simulink model "gyroscope_temps_reel"  (R2013a)
settings: Solver=ode3  StartTime=0.0  StopTime=inf  FixedStep=Ts  RelTol=1e-3
values from neighbouring files (symbols this model uses):
  Aobs2 = A2-H2*C2    [speed_w1_estimation.m]
  Bobs2 = [B2 H2]    [speed_w1_estimation.m]
  Cobs2 = [0 1]    [speed_w1_estimation.m]
  Dobs2 = zeros(1,2)    [speed_w1_estimation.m]
  Te = Ts    [speed_w1_estimation.m]
undefined symbols (not defined in the file or in its folder): C0, Kp, Standard_Devices, UDP_Protocol
libraries: etargetslib x13, simulink x2, rtwinlib x2
settings Model: SimulationMode=external  ExtModeTrigDuration=100000  Creator=dumonjon  LastModifiedBy=khennouh
settings DataIOCC: LimitDataPoints=off  SaveFormat=StructureWithTime  SignalLoggingSaveFormat=ModelDataLogs  SaveOutput=off  SignalLogging=off  SaveTime=off
settings OptimizationCC: ExpressionDepthLimit=2147483647  InitFltsAndDblsToZero=on
settings DebuggingCC: FcnCallInpInsideContextMsg=UseLocalSettings  StrictBusMsg=Warning
settings SFSimCC: SimParseCustomCode=off
settings RTWCC: SystemTargetFile=rtwin.tlc  TemplateMakefile=rtwin.tmf  Description=Real-Time Windows Target  ProcessScript=rtwin_make_rtw_hook
settings TargetCC: CodeReplacementLibrary=ANSI_C  IsPILTarget=off  ModelReferenceCompliant=off  CompOptLevelCompliant=off  EnableShiftOperators=on

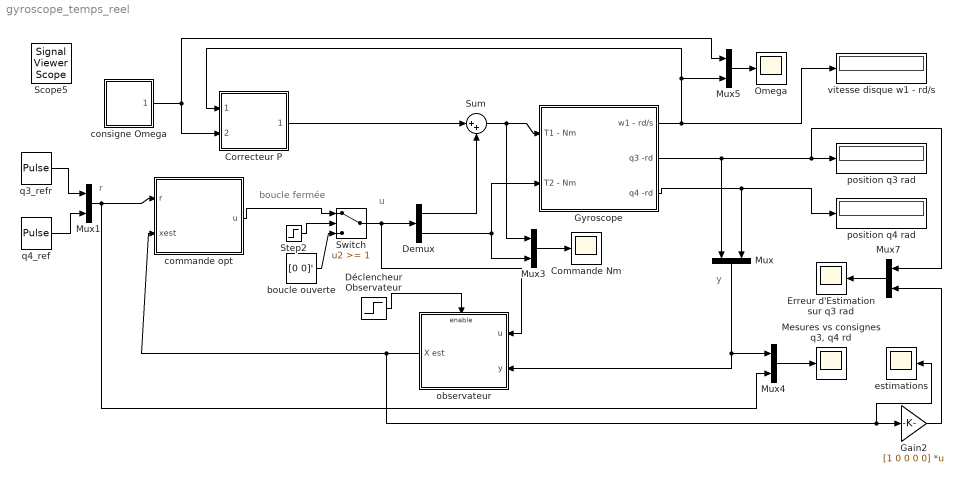
== system gyroscope_temps_reel ==
  note: u
  note: r
  note: y
  note: boucle fermée
  Commande Nm : Scope
      settings: TimeRange=70  YMin=-0.2  YMax=0.5  SaveName=commande
  Correcteur P : Subsystem
  Demux : Demux  Outputs=2
  Déclencheur Observateur : Step  SampleTime=0
  Erreur d'Estimation sur q3 rad : Scope
      settings: TimeRange=70  YMin=-0.6000000000000001  YMax=0.8  SaveName=theta3
  Gain2 : Gain  Gain=[1 0 0 0 0]  Multiplication=Matrix(K*u) (u vector)
  Gyroscope : Subsystem
  "Mesures vs consignes q3, q4 rd" : Scope
      settings: TimeRange=70  YMin=-0.35  YMax=0.35  SaveName=consigne
  Mux{,1,3..5,7} (6 alike) : Mux  Inputs=2
  Omega : Scope
      settings: TimeRange=60  YMin=0  YMax=60  SaveName=omega
  Step2 : Step  Time=15  SampleTime=0
  Sum : Sum  Inputs=|++
  Switch : Switch  Threshold=1
  boucle ouverte : Constant  Value=[0 0]'
  commande opt : Subsystem
  consigne Omega : Subsystem  mask{Omega=42}
  estimations : Scope
      settings: TimeRange=70  YMin=-1.5  YMax=1  SaveName=estimations
  observateur : Subsystem
  position q3 rad : Display
  position q4 rad : Display
  q3_refr : DiscretePulseGenerator  PulseType=Time based  Amplitude=10*pi/180  Period=20  PulseWidth=50  PhaseDelay=20
  q4_ref : DiscretePulseGenerator  PulseType=Time based  Amplitude=10*pi/180  Period=20  PulseWidth=50  PhaseDelay=25
  vitesse disque w1 - rd/s : Display
  Scope5 : SignalViewerScope  IOType=viewer  RefreshTime=0.035000
  wires:
  consigne Omega/1(Cw1 rd/s) -> Correcteur P/2(Cw1 rd/s), Mux5/1
  Demux/2 -> Mux3/2, Gyroscope/2(T2 - Nm)
  Sum/1 -> Gyroscope/1(T1 - Nm), Mux3/1
  Gyroscope/2(q3 -rd) -> Mux/1, position q3 rad/1, Mux7/1
  Gyroscope/3(q4 -rd) -> Mux/2, position q4 rad/1
  Mux/1 -> Mux4/1, observateur/2(y)
  q4_ref/1 -> Mux1/2
  Switch/1 -> Demux/1, observateur/1(u)
  commande opt/1(u) -> Switch/1
  boucle ouverte/1 -> Switch/3
  Mux3/1 -> Commande Nm/1
  Correcteur P/1(T1 Nm) -> Sum/1
  observateur/1(X est) -> Gain2/1, estimations/1, commande opt/2(xest)
  Step2/1 -> Switch/2
  q3_refr/1 -> Mux1/1
  Mux4/1 -> "Mesures vs consignes q3, q4 rd"/1
  Demux/1 -> Sum/2
  Mux5/1 -> Omega/1
  Gyroscope/1(w1 - rd/s) -> vitesse disque w1 - rd/s/1, Correcteur P/1(w1 rd/s), Mux5/2
  Mux7/1 -> Erreur d'Estimation sur q3 rad/1
  Gain2/1 -> Mux7/2
  Déclencheur Observateur/1 -> observateur/Enable
  Mux1/1 -> commande opt/1(r), Mux4/2

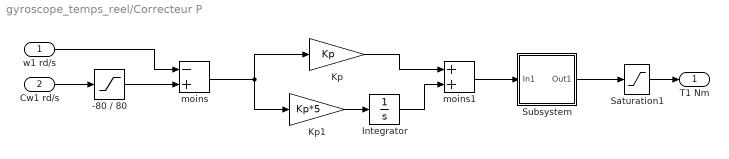
== system gyroscope_temps_reel/Correcteur P ==
  w1 rd/s : Inport
  Cw1 rd/s : Inport  Port=2
  -80 / 80 : Saturate  UpperLimit=80  LowerLimit=-80
  Integrator : Integrator
  Kp : Gain  Gain=Kp
  Kp1 : Gain  Gain=Kp*5
  Saturation1 : Saturate  UpperLimit=0.2  LowerLimit=-0.2
  Subsystem : Subsystem
  moins : Sum  Inputs=-+
  moins1 : Sum
  T1 Nm : Outport
  wires:
  -80 / 80/1 -> moins/2
  Cw1 rd/s/1 -> -80 / 80/1
  w1 rd/s/1 -> moins/1
  Saturation1/1 -> T1 Nm/1
  Kp1/1 -> Integrator/1
  moins1/1 -> Subsystem/1(In1)
  Integrator/1 -> moins1/2
  Kp/1 -> moins1/1
  moins/1 -> Kp/1, Kp1/1
  Subsystem/1(Out1) -> Saturation1/1

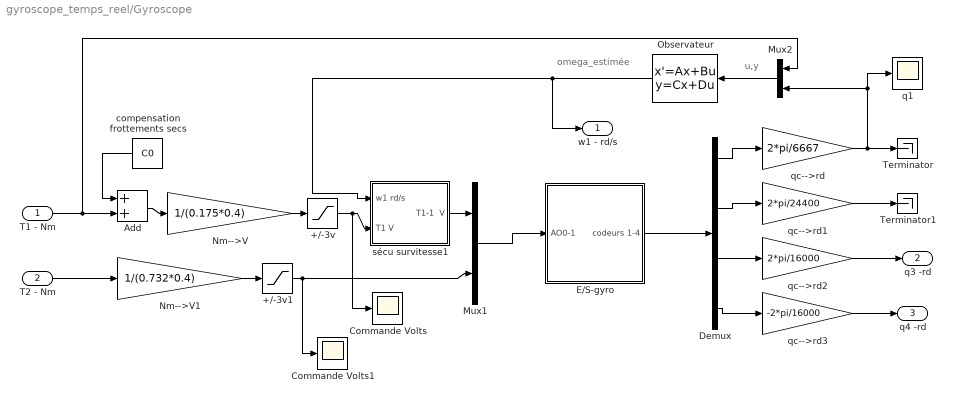
== system gyroscope_temps_reel/Gyroscope ==
  note: omega_estimée
  note: u,y
  T1 - Nm : Inport
  T2 - Nm : Inport  Port=2
  +/-3v : Saturate  UpperLimit=5  LowerLimit=-5
  +/-3v1 : Saturate  UpperLimit=+10  LowerLimit=-10
  Add : Sum
  Commande Volts : Scope
      settings: TimeRange=40  YMin=-3  YMax=3  SaveName=commande1
  Commande Volts1 : Scope
      settings: TimeRange=40  YMin=-4  YMax=4  SaveName=commande2
  Demux : Demux
  E/S-gyro : Subsystem
  Mux1 : Mux  Inputs=2
  Mux2 : Mux  Inputs=2
  Nm-->V : Gain  Gain=1/(0.175*0.4)
  Nm-->V1 : Gain  Gain=1/(0.732*0.4)
  Observateur : StateSpace  A=Aobs2  B=Bobs2  C=Cobs2  D=Dobs2
  Terminator : Terminator
  Terminator1 : Terminator
  compensation frottements secs : Constant  Value=C0
  q1 : Scope
      settings: TimeRange=80  YMin=2431.26  YMax=2687.18  SaveName=vitesses4
  qc-->rd : Gain  Gain=2*pi/6667
  qc-->rd1 : Gain  Gain=2*pi/24400
  qc-->rd2 : Gain  Gain=2*pi/16000
  qc-->rd3 : Gain  Gain=-2*pi/16000
  sécu survitesse1 : Subsystem
  w1 - rd/s : Outport
  q3 -rd : Outport  Port=2
  q4 -rd : Outport  Port=3
  wires:
  Demux/1 -> qc-->rd/1
  Demux/2 -> qc-->rd1/1
  Demux/3 -> qc-->rd2/1
  Demux/4 -> qc-->rd3/1
  Nm-->V/1 -> +/-3v/1
  Nm-->V1/1 -> +/-3v1/1
  qc-->rd/1 -> q1/1, Mux2/2, Terminator/1
  qc-->rd2/1 -> q3 -rd/1
  +/-3v/1 -> sécu survitesse1/2(T1 V), Commande Volts/1
  sécu survitesse1/1(T1-1  V) -> Mux1/1
  qc-->rd1/1 -> Terminator1/1
  T2 - Nm/1 -> Nm-->V1/1
  compensation frottements secs/1 -> Add/1
  T1 - Nm/1 -> Add/2, Mux2/1
  Add/1 -> Nm-->V/1
  +/-3v1/1 -> Mux1/2, Commande Volts1/1
  Mux2/1 -> Observateur/1
  Observateur/1 -> w1 - rd/s/1, sécu survitesse1/1(w1 rd/s)
  qc-->rd3/1 -> q4 -rd/1
  E/S-gyro/1(codeurs 1-4) -> Demux/1
  Mux1/1 -> E/S-gyro/1("AO0-1 ")

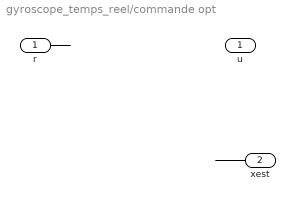
== system gyroscope_temps_reel/commande opt ==
  r : Inport
  xest : Inport  Port=2
  u : Outport
  wires:
  xest/1 -> ?
  r/1 -> ?

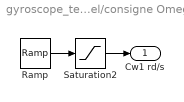
== system gyroscope_temps_reel/consigne Omega ==
  Ramp : simulink/Sources/Ramp  SystemSampleTime=-1  slope=5  start=0  X0=0
  Saturation2 : Saturate  UpperLimit=Omega  LowerLimit=0
  Cw1 rd/s : Outport
  wires:
  Ramp/1 -> Saturation2/1
  Saturation2/1 -> Cw1 rd/s/1

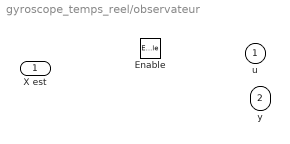
== system gyroscope_temps_reel/observateur ==
  u : Inport
  y : Inport  Port=2
  Enable : EnablePort
  X est : Outport

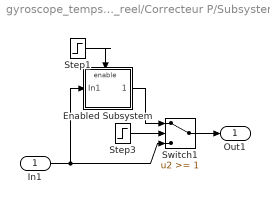
== system gyroscope_temps_reel/Correcteur P/Subsystem ==
  In1 : Inport
  Enabled Subsystem : Subsystem  TreatAsAtomicUnit=on
  Step1 : Step  Time=12  SampleTime=0
  Step3 : Step  Time=14  SampleTime=0
  Switch1 : Switch  Threshold=1
  Out1 : Outport
  wires:
  Step3/1 -> Switch1/2
  Enabled Subsystem/1(Out1) -> Switch1/1
  In1/1 -> Switch1/3, Enabled Subsystem/1(In1)
  Step1/1 -> Enabled Subsystem/Enable
  Switch1/1 -> Out1/1

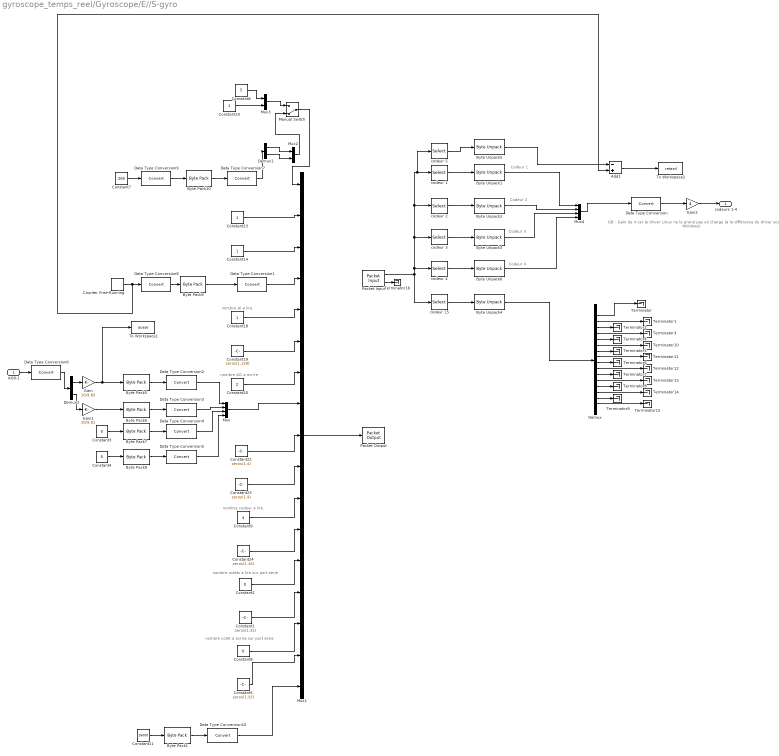
== system gyroscope_temps_reel/Gyroscope/E//S-gyro ==
  note: Codeur 4
  note: Codeur 3
  note: Codeur 2
  note: Codeur 1
  note: GB : Gain de 4 car le driver Linux
      |  ne le prend pas en charge
      | (à la différence du driver sous Windows)
  note: nombre AO a ecrire
  note: nombre AI a lire
  note: nombre codeur a lire
  note: nombre octets a lire sur port serie
  note: nombre octet a ecrire sur port serie
  "AO0-1 " : Inport
  Add1 : Sum  Inputs=-+
  Byte Pack1 : etargetslib/Byte Pack  datatypes={'uint32'}  byteAlign=1
  Byte Pack10 : etargetslib/Byte Pack  datatypes={'int16'}  byteAlign=1
  Byte Pack{5..8} (4 alike) : etargetslib/Byte Pack  datatypes={'double'}  byteAlign=1
  Byte Pack9 : etargetslib/Byte Pack  datatypes={'uint32'}  byteAlign=1
  Byte Unpack{1..3,6} (4 alike) : etargetslib/Byte Unpack  dimensions={[1]}  datatypes={'int32'}  byteAlign=4
  Byte Unpack4 : etargetslib/Byte Unpack  dimensions={[16]}  datatypes={'double'}  byteAlign=4
  Byte Unpack5 : etargetslib/Byte Unpack  dimensions={[1]}  datatypes={'uint32'}  byteAlign=4
  Constant1 : Constant  Value=zeros(1,32)
  Constant{10,13..14,18} (4 alike) : Constant
  Constant11 : Constant  Value=16000  OutDataTypeStr=uint32
  Constant19 : Constant  Value=zeros(1,128)
  Constant2 : Constant  Value=0
  Constant20 : Constant  Value=2  OutDataTypeStr=Inherit: Inherit via back propagation
  Constant22 : Constant  Value=zeros(1,4)
  Constant23 : Constant  Value=zeros(1,4)
  Constant24 : Constant  Value=zeros(1,16)
  Constant3 : Constant  Value=0  OutDataTypeStr=double
  Constant4 : Constant  Value=0  OutDataTypeStr=double
  Constant5 : Constant  Value=zeros(1,32)
  Constant6 : Constant  Value=0
  Constant7 : Constant  Value=265
  Constant8 : Constant  Value=5
  Constant9 : Constant  Value=4
  Counter Free-Running : simulink/Sources/Counter Free-Running  NumBits=32  tsamp=-1
  Data Type Conversion{,1..10} (11 alike) : DataTypeConversion
  Demux : Demux  Outputs=16
  Demux1 : Demux  Outputs=2
  Demux2 : Demux  Outputs=2
  Gain : Gain  Gain=10/9.83
  Gain1 : Gain  Gain=10/9.81
  Gain2 : Gain  Gain=4
  Manual Switch : ManualSwitch  CurrentSetting=0
  Mux : Mux
  Mux1 : Mux  Inputs=17
  Mux2 : Mux  Inputs=2
  Mux3 : Mux  Inputs=2
  Mux4 : Mux
  Packet Input : rtwinlib/Packet Input  SampleTime=Te  MaxMissedTicks=10  ShowMissedTicks=on  YieldWhenWaiting=off  DrvName=Standard_Devices/UDP_Protocol  DrvAddress=9930  DrvOptions=[3232235522 9930]  PacketSize=265  DataTypes='265*uint8'  ShowReady=off  ShowError=off  PacketID=1  ByteOrder=1  ShowTimestamp=off
      settings: AttributesFormatString=Standard Devices\nUDP Protocol [26CAh]
  Packet Output : rtwinlib/Packet Output  SampleTime=Te  MaxMissedTicks=10  ShowMissedTicks=off  YieldWhenWaiting=off  DrvName=Standard_Devices/UDP_Protocol  DrvAddress=9930  DrvOptions=[3232235522 9930]  PacketSize=265  DataTypes='265*uint8'  ShowReady=off  ShowError=off  PacketID=1  ByteOrder=1  InitialValue=[]  FinalValue=[]
      settings: AttributesFormatString=Standard Devices\nUDP Protocol [26CAh]
  Terminator{,1..16} (17 alike) : Terminator
  To Workspace1 : ToWorkspace  VariableName=aoser  SampleTime=-1  SaveFormat=Structure With Time
  To Workspace2 : ToWorkspace  VariableName=retard  SampleTime=-1  SaveFormat=Structure With Time
  codeur 1 : Selector  InputPortWidth=265  IndexOptions=Index vector (dialog)  Indices=[180 181 182 183]  OutputSizes=1
  codeur 15 : Selector  InputPortWidth=265  IndexOptions=Index vector (dialog)  Indices=[10:137]  OutputSizes=1
  codeur 2 : Selector  InputPortWidth=265  IndexOptions=Index vector (dialog)  Indices=[184 185 186 187]  OutputSizes=1
  codeur 3 : Selector  InputPortWidth=265  IndexOptions=Index vector (dialog)  Indices=[188 189 190 191]  OutputSizes=1
  codeur 4 : Selector  InputPortWidth=265  IndexOptions=Index vector (dialog)  Indices=[192 193 194 195]  OutputSizes=1
  codeur 5 : Selector  InputPortWidth=265  IndexOptions=Index vector (dialog)  Indices=[5 6 7 8]  OutputSizes=1
  codeurs 1-4 : Outport
  wires:
  Constant13/1 -> Mux1/2
  Constant14/1 -> Mux1/3
  Constant18/1 -> Mux1/5
  Constant19/1 -> Mux1/6
  Constant20/1 -> Mux1/7
  Mux/1 -> Mux1/8
  Constant22/1 -> Mux1/9
  Constant23/1 -> Mux1/10
  Constant9/1 -> Mux1/11
  Constant24/1 -> Mux1/12
  Mux1/1 -> Packet Output/1
  Data Type Conversion5/1 -> Mux/4
  Data Type Conversion4/1 -> Mux/3
  Constant3/1 -> Byte Pack7/1
  Constant4/1 -> Byte Pack8/1
  Data Type Conversion1/1 -> Mux1/4
  Byte Pack8/1 -> Data Type Conversion5/1
  Byte Pack7/1 -> Data Type Conversion4/1
  Data Type Conversion2/1 -> Mux/1
  Byte Pack5/1 -> Data Type Conversion2/1
  Data Type Conversion3/1 -> Mux/2
  Byte Pack6/1 -> Data Type Conversion3/1
  codeur 15/1 -> Byte Unpack4/1
  Constant1/1 -> Mux1/14
  Constant2/1 -> Mux1/13
  Constant6/1 -> Mux1/15
  Constant7/1 -> Data Type Conversion9/1
  Byte Pack10/1 -> Data Type Conversion7/1
  Packet Input/1 -> codeur 5/1, codeur 1/1, codeur 2/1, codeur 3/1, codeur 4/1, codeur 15/1
  Data Type Conversion7/1 -> Demux1/1
  Manual Switch/1 -> Mux1/1
  Mux3/1 -> Manual Switch/1
  Constant10/1 -> Mux3/2
  Constant8/1 -> Mux3/1
  Mux4/1 -> Data Type Conversion/1
  "AO0-1 "/1 -> Data Type Conversion6/1
  Constant5/1 -> Mux1/16
  Data Type Conversion/1 -> Gain2/1
  Data Type Conversion6/1 -> Demux2/1
  Data Type Conversion8/1 -> Byte Pack9/1
  Demux2/2 -> Gain1/1
  Demux2/1 -> Gain/1
  Gain/1 -> To Workspace1/1, Byte Pack5/1
  Gain1/1 -> Byte Pack6/1
  Mux2/1 -> Manual Switch/2
  Data Type Conversion9/1 -> Byte Pack10/1
  codeur 1/1 -> Byte Unpack1/1
  Byte Unpack1/1 -> Mux4/1
  codeur 2/1 -> Byte Unpack2/1
  codeur 3/1 -> Byte Unpack3/1
  codeur 4/1 -> Byte Unpack6/1
  Byte Unpack6/1 -> Mux4/4
  Byte Unpack3/1 -> Mux4/3
  Byte Unpack2/1 -> Mux4/2
  Gain2/1 -> codeurs 1-4/1
  Byte Unpack4/1 -> Demux/1
  Demux/2 -> Terminator1/1
  Demux/3 -> Terminator2/1
  Demux/4 -> Terminator3/1
  Demux/8 -> Terminator11/1
  Demux/6 -> Terminator10/1
  Demux/5 -> Terminator4/1
  Demux/9 -> Terminator6/1
  Demux/7 -> Terminator5/1
  Demux/10 -> Terminator12/1
  Demux/11 -> Terminator7/1
  Demux/13 -> Terminator8/1
  Demux/15 -> Terminator9/1
  Demux/12 -> Terminator13/1
  Demux/14 -> Terminator14/1
  Demux/16 -> Terminator15/1
  codeur 5/1 -> Byte Unpack5/1
  Byte Unpack5/1 -> Add1/1
  Byte Pack9/1 -> Data Type Conversion1/1
  Counter Free-Running/1 -> Add1/2, Data Type Conversion8/1
  Demux/1 -> Terminator/1
  Constant11/1 -> Byte Pack1/1
  Byte Pack1/1 -> Data Type Conversion10/1
  Data Type Conversion10/1 -> Mux1/17
  Add1/1 -> To Workspace2/1
  Demux1/2 -> Mux2/2
  Demux1/1 -> Mux2/1
  Packet Input/2 -> Terminator16/1

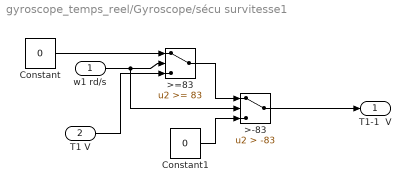
== system gyroscope_temps_reel/Gyroscope/sécu survitesse1 ==
  w1 rd/s : Inport
  T1 V : Inport  Port=2
  >-83 : Switch  Criteria=u2 > Threshold  Threshold=-83
  >=83 : Switch  Threshold=83
  Constant : Constant  Value=0
  Constant1 : Constant  Value=0
  T1-1  V : Outport
  wires:
  >-83/1 -> T1-1  V/1
  Constant1/1 -> >-83/3
  T1 V/1 -> >=83/3
  >=83/1 -> >-83/1
  w1 rd/s/1 -> >-83/2, >=83/2
  Constant/1 -> >=83/1

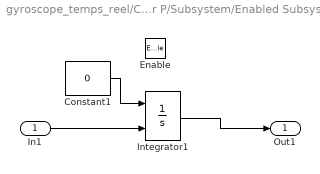
== system gyroscope_temps_reel/Correcteur P/Subsystem/Enabled Subsystem ==
  In1 : Inport
  Enable : EnablePort
  Constant1 : Constant  Value=0
  Integrator1 : Integrator  InitialConditionSource=external
  Out1 : Outport
  wires:
  In1/1 -> Integrator1/2
  Integrator1/1 -> Out1/1
  Constant1/1 -> Integrator1/1
